simulink model "downsample_tut1"  (Simulink 5.0)
settings: Solver=FixedStepDiscrete  StartTime=0.0  StopTime=10.0  RelTol=1e-3
libraries: dspsigops x1, dspxfrm3 x1, dspsrcs4 x1
settings Model: CovMetricSettings=d  Creator=ckamachi  LastModifiedBy=ckamachi  ExtModeTrigMode=oneshot  ExtModeArmWhenConnect=off  LimitDataPoints=off  BlockReductionOpt=off  BooleanDataType=off

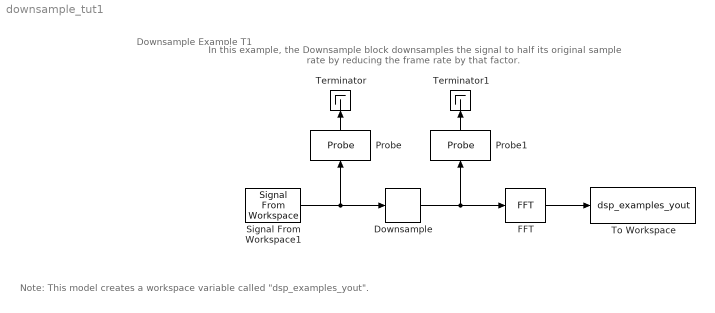
== system downsample_tut1 ==
  note: Downsample Example T1
  note: In this example, the Downsample block downsamples the signal to half
      | its original sample rate by reducing the frame rate by that factor.
  note: Note: This model creates a workspace variable called "dsp_examples_yout".
  Downsample : dspsigops/Downsample  N=2  phase=0  ic=0  smode=Allow multirate  fmode=Maintain input frame size
  FFT : dspxfrm3/FFT  CompMethod=Table lookup  TableOpt=Speed  BitRevOrder=off
  Probe : Probe  Orientation=up  ProbeWidth=off  ProbeComplexSignal=off
  Probe1 : Probe  Orientation=up  ProbeWidth=off  ProbeComplexSignal=off
  Signal From Workspace1 : dspsrcs4/Signal From Workspace  X=1:1000  Ts=0.125  nsamps=8  OutputAfterFinalValue=Setting to zero
  Terminator : Terminator
      settings: Orientation=up
  Terminator1 : Terminator
      settings: Orientation=up
  To Workspace : ToWorkspace  VariableName=dsp_examples_yout  SampleTime=-1  SaveFormat=Array
  wires:
  FFT/1 -> To Workspace/1
  Signal From Workspace1/1 -> Downsample/1, Probe/1
  Downsample/1 -> FFT/1, Probe1/1
  Probe/1 -> Terminator/1
  Probe1/1 -> Terminator1/1
